simulink model "ssr_dev"  (R2020b)
settings: Solver=VariableStepAuto  StartTime=0.0  StopTime=10.0  RelTol=1e-3
libraries: hdlsllib x17
settings Model: Creator=LDM  LastModifiedBy=ckb13136

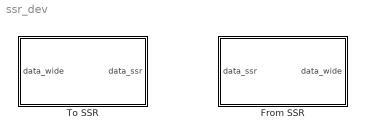
== system ssr_dev ==
  From SSR : Subsystem
  To SSR : Subsystem  mask{w=3, ssr=16}
      mask init:
      | top_block = gcb;
      | block_names = find_system(top_block, 'LookUnderMasks','on', 'SearchDepth','1');
      | 
      | in_block = sprintf('%s/data_wide', top_block);
      | out_block = sprintf('%s/data_ssr', top_block);
      | bit_slice = sprintf('%s/Bit Slice 0', top_block);
      | 
      | keep_blocks = {top_block, in_block, out_block, bit_slice};
      | 
      | for i = 1:length(block_names)
      |     if ~ismember(block_names{i}, keep_blocks)
      |         delete_block(block_names{i});
      |     end
      | end
      | delete_line(find_system(top_block,'LookUnderMasks', 'all','SearchDepth', '1', 'FindAll','on','type','line'));
      | 
      | % Add Bit Slice Blocks
      | pos = get_param(bit_slice, 'position');
      | set_param(bit_slice, 'lidx', num2str(w-1));
      | set_param(bit_slice, 'ridx', num2str(0));
      | for slice = 2:ssr
      |     new_block = sprintf('%s%d', bit_slice(1:end-1), (slice-1));
      |     add_block(bit_slice, new_block);
      |     new_pos = pos + ([0 60 0 60] * (slice-1));
      |     set_param(new_block, 'position', new_pos);
      |     set_param(new_block, 'lidx', num2str(slice*w-1));
      |     set_param(new_block, 'ridx', num2str((slice-1)*w));
      | end
      | 
      | % Add the Mux
      | mux_block = sprintf('%s/mux', top_block);
      | add_block('simulink/Signal Routing/Mux', mux_block);
      | set_param(mux_block, 'Inputs', num2str(ssr));
      | mux_position = new_pos + [125 0 70 0];
      | mux_position(2) = pos(2);
      | set_param(mux_block, 'position', mux_position);
      | 
      | % Add Reshape
      | rshp_block = sprintf('%s/reshape', top_block);
      | add_block('simulink/Math Operations/Reshape', rshp_block);
      | set_param(rshp_block, 'OutputDimensionality', 'Row vector (2-D)');
      | rshp_position = new_pos + [180 0 180 0];
      | 
      | % Reposition Input and Outputs
      | out_position = get_param(out_block, 'position');
      | height = out_position(4) - out_position(2);
      | width = out_position(3) - out_position(1);
      | middle_h = (mux_position(4) - mux_position(2))/2 + mux_position(2);
      | out_position = [mux_position(1) + 175, middle_h - height/2, mux_position(1) + 175 + width, middle_h + height/2];
      | set_param(out_block, 'position', out_position);
      | 
      | in_position = [mux_position(1) - 300, middle_h - height/2, mux_position(1) - 300 + width, middle_h + height/2];
      | set_param(in_block, 'position', in_position);
      | 
      | rshp_position(2) = middle_h - 25;
      | rshp_position(4) = middle_h + 25;
      | set_param(rshp_block, 'position', rshp_position);
      | 
      | % Connect Ports
      | for slice = 1:ssr
      |     add_line(top_block,'data_wide/1',sprintf('Bit Slice %d/1',slice-1));
      |     add_line(top_block,sprintf('Bit Slice %d/1',(slice-1)),sprintf('mux/%d', slice));
      | end
      | add_line(top_block,'mux/1','reshape/1');
      | add_line(top_block,'reshape/1','data_ssr/1');

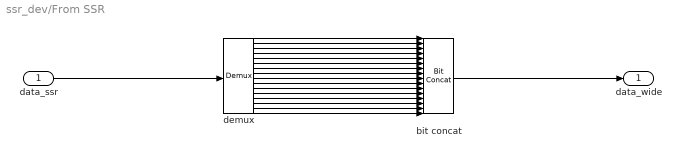
== system ssr_dev/From SSR ==
  data_ssr : Inport
  bit concat : hdlsllib/Logic and Bit Operations/Bit Concat  numInputs=16
  demux : Demux  Outputs=16
  data_wide : Outport
  wires:
  demux/1 -> bit concat/1
  demux/2 -> bit concat/2
  demux/3 -> bit concat/3
  demux/4 -> bit concat/4
  demux/5 -> bit concat/5
  demux/6 -> bit concat/6
  demux/7 -> bit concat/7
  demux/8 -> bit concat/8
  demux/9 -> bit concat/9
  demux/10 -> bit concat/10
  demux/11 -> bit concat/11
  demux/12 -> bit concat/12
  demux/13 -> bit concat/13
  demux/14 -> bit concat/14
  demux/15 -> bit concat/15
  demux/16 -> bit concat/16
  data_ssr/1 -> demux/1
  bit concat/1 -> data_wide/1

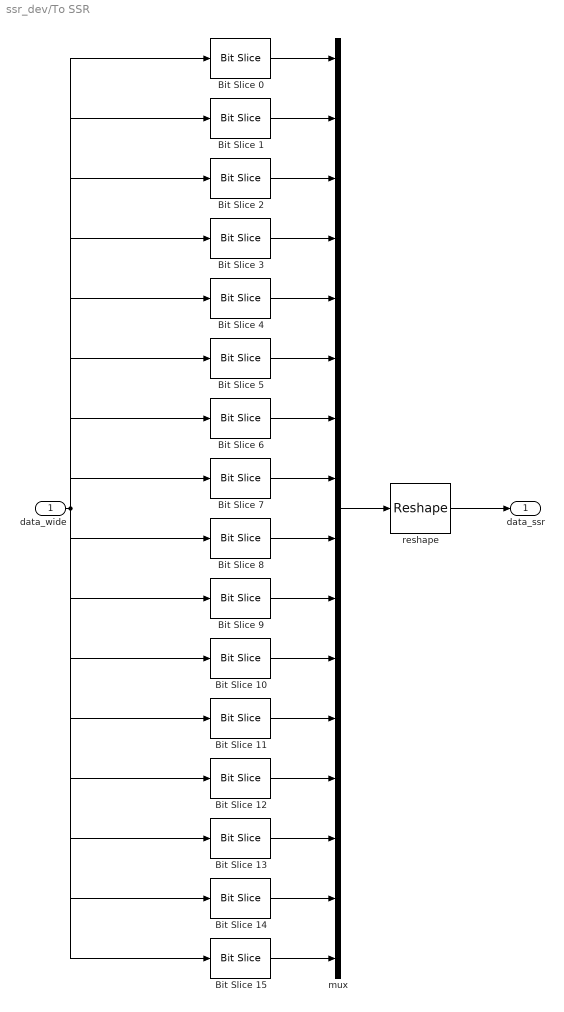
== system ssr_dev/To SSR ==
  data_wide : Inport
  Bit Slice 0 : hdlsllib/Logic and Bit Operations/Bit Slice  lidx=2  ridx=0
      settings: SourceProductBaseCode=SL
  Bit Slice 1 : hdlsllib/Logic and Bit Operations/Bit Slice  lidx=5  ridx=3
      settings: SourceProductBaseCode=SL
  Bit Slice 10 : hdlsllib/Logic and Bit Operations/Bit Slice  lidx=32  ridx=30
      settings: SourceProductBaseCode=SL
  Bit Slice 11 : hdlsllib/Logic and Bit Operations/Bit Slice  lidx=35  ridx=33
      settings: SourceProductBaseCode=SL
  Bit Slice 12 : hdlsllib/Logic and Bit Operations/Bit Slice  lidx=38  ridx=36
      settings: SourceProductBaseCode=SL
  Bit Slice 13 : hdlsllib/Logic and Bit Operations/Bit Slice  lidx=41  ridx=39
      settings: SourceProductBaseCode=SL
  Bit Slice 14 : hdlsllib/Logic and Bit Operations/Bit Slice  lidx=44  ridx=42
      settings: SourceProductBaseCode=SL
  Bit Slice 15 : hdlsllib/Logic and Bit Operations/Bit Slice  lidx=47  ridx=45
      settings: SourceProductBaseCode=SL
  Bit Slice 2 : hdlsllib/Logic and Bit Operations/Bit Slice  lidx=8  ridx=6
      settings: SourceProductBaseCode=SL
  Bit Slice 3 : hdlsllib/Logic and Bit Operations/Bit Slice  lidx=11  ridx=9
      settings: SourceProductBaseCode=SL
  Bit Slice 4 : hdlsllib/Logic and Bit Operations/Bit Slice  lidx=14  ridx=12
      settings: SourceProductBaseCode=SL
  Bit Slice 5 : hdlsllib/Logic and Bit Operations/Bit Slice  lidx=17  ridx=15
      settings: SourceProductBaseCode=SL
  Bit Slice 6 : hdlsllib/Logic and Bit Operations/Bit Slice  lidx=20  ridx=18
      settings: SourceProductBaseCode=SL
  Bit Slice 7 : hdlsllib/Logic and Bit Operations/Bit Slice  lidx=23  ridx=21
      settings: SourceProductBaseCode=SL
  Bit Slice 8 : hdlsllib/Logic and Bit Operations/Bit Slice  lidx=26  ridx=24
      settings: SourceProductBaseCode=SL
  Bit Slice 9 : hdlsllib/Logic and Bit Operations/Bit Slice  lidx=29  ridx=27
      settings: SourceProductBaseCode=SL
  mux : Mux  Inputs=16
  reshape : Reshape  OutputDimensionality=Row vector (2-D)
  data_ssr : Outport
  wires:
  data_wide/1 -> Bit Slice 0/1, Bit Slice 1/1, Bit Slice 2/1, Bit Slice 3/1, Bit Slice 4/1, Bit Slice 5/1, Bit Slice 6/1, Bit Slice 7/1, Bit Slice 8/1, Bit Slice 9/1, Bit Slice 10/1, Bit Slice 11/1, Bit Slice 12/1, Bit Slice 13/1, Bit Slice 14/1, Bit Slice 15/1
  Bit Slice 0/1 -> mux/1
  Bit Slice 1/1 -> mux/2
  Bit Slice 2/1 -> mux/3
  Bit Slice 3/1 -> mux/4
  Bit Slice 4/1 -> mux/5
  Bit Slice 5/1 -> mux/6
  Bit Slice 6/1 -> mux/7
  Bit Slice 7/1 -> mux/8
  Bit Slice 8/1 -> mux/9
  Bit Slice 9/1 -> mux/10
  Bit Slice 10/1 -> mux/11
  Bit Slice 11/1 -> mux/12
  Bit Slice 12/1 -> mux/13
  Bit Slice 13/1 -> mux/14
  Bit Slice 14/1 -> mux/15
  Bit Slice 15/1 -> mux/16
  mux/1 -> reshape/1
  reshape/1 -> data_ssr/1
